simulink model "RobotModel6"  (R2025b)
settings: Solver=VariableStepAuto  StartTime=0.0  StopTime=100  RelTol=0.01  AbsTol=0.01  EnableMultiTasking=on
values from neighbouring files (symbols this model uses):
  waypoints = [R*cos(theta)+5, R*sin(theta)]    [init_waypoints.m]
undefined symbols (not defined in the file or in its folder): X, Y, Z
libraries: sm_lib x76, nesl_utility x37, slpidlib x2, robotalgslib x1, sharedtransform x1
(part 4 of 4)

== system RobotModel6/Subsystem5 ==
  In2 : Inport
  wR_cmd : Inport  Port=2
  PID Controller : slpidlib/PID Controller  Controller=PID  Form=Parallel  TimeDomain=Continuous-time  UseExternalTs=off  SampleTime=-1  IntegratorMethod=Forward Euler  FilterMethod=Forward Euler  ControllerParametersSource=internal  P=5  I=0  UseKiTs=off  D=0  UseExternalDerivativeSource=off  N=100  UseFilter=on  TunerSelectOption=Transfer Function Based (PID Tuner App)  InitialConditionSource=internal  InitialConditionForIntegrator=0  InitialConditionForFilter=0  DifferentiatorICPrevScaledInput=0  ExternalReset=none  TrackingMode=off  Kt=1  LimitOutput=off  SatLimitsSource=internal  UpperSaturationLimit=inf  LowerSaturationLimit=-inf  LinearizeAsGain=on  AntiWindupMode=none  Kb=1  LimitIntegrator=off  UpperIntegratorSaturationLimit=inf  LowerIntegratorSaturationLimit=-inf  POutMin=[]  POutMax=[]  IOutMin=[]  IOutMax=[]  DOutMin=[]  DOutMax=[]  NOutMin=[]  NOutMax=[]  SumOutMin=[]  SumOutMax=[]  SaturationOutMin=[]  SaturationOutMax=[]  PParamMin=[]  PParamMax=[]  IParamMin=[]  IParamMax=[]  DParamMin=[]  DParamMax=[]  NParamMin=[]  NParamMax=[]  KbParamMin=[]  KbParamMax=[]  KtParamMin=[]  KtParamMax=[]  KbOutMin=[]  KbOutMax=[]  KtOutMin=[]  KtOutMax=[]  IntegratorOutMin=[]  IntegratorOutMax=[]  FilterOutMin=[]  FilterOutMax=[]  SumI1OutMin=[]  SumI1OutMax=[]  SumI2OutMin=[]  SumI2OutMax=[]  SumI3OutMin=[]  SumI3OutMax=[]  SumI4OutMin=[]  SumI4OutMax=[]  SumDOutMin=[]  SumDOutMax=[]  DifferentiatorOutMin=[]  DifferentiatorOutMax=[]  FilterDiffOutCoefMin=[]  FilterDiffOutCoefMax=[]  ReciprocalOutMin=[]  ReciprocalOutMax=[]  SumDenOutMin=[]  SumDenOutMax=[]  SumNumOutMin=[]  SumNumOutMax=[]  DivideOutMin=[]  DivideOutMax=[]  UdiffTsProdOutMin=[]  UdiffTsProdOutMax=[]  NTsProdOutMin=[]  NTsProdOutMax=[]  UintegralTsProdOutMin=[]  UintegralTsProdOutMax=[]  UngainTsProdOutMin=[]  UngainTsProdOutMax=[]  ClampingZeroOutDataTypeStr=Inherit: Inherit via back propagation  ClampingZeroOutMin=[]  ClampingZeroOutMax=[]  FilterDenConstantOutDataTypeStr=Inherit: Inherit via back propagation  FilterDenConstantOutMin=[]  FilterDenConstantOutMax=[]  PCopyOutDataTypeStr=Inherit: Inherit via back propagation  PCopyOutMin=[]  PCopyOutMax=[]  NCopyOutDataTypeStr=Inherit: Inherit via back propagation  NCopyOutMin=[]  NCopyOutMax=[]  IntegratorContinuousStateAttributes=''  IntegratorStateMustResolveToSignalObject=off  IntegratorRTWStateStorageClass=Auto  FilterContinuousStateAttributes=''  FilterStateMustResolveToSignalObject=off  FilterRTWStateStorageClass=Auto  ParallelPVariant=InternalParameters  IdealPVariant=Disabled  IVariant=InternalParameters  DVariant=InternalParameters  IntegratorVariant=Continuous  SatVariant=Disabled  AWVariant=Passthrough  PCopyVariant=Disabled  TRVariant=Disabled  FdbkBlocksVariant=Forward  IdealPFdbkVariant=Disabled  SatFdbkVariant=Disabled  DerivativeFilterVariant=ContFilter  NVariant=InternalParameters  NCopyVariant=Disabled  FilterICVariant=InternalICsFilter  IntegratorICVariant=InternalICs  ExternalResetVariant=Disabled  TRSumVariant=Passthrough  SumFdbkVariant=Disabled  SumVariant=Sum_PID  TsampFilterVariant=InternalTs  TsampNgainVariant=Passthrough  TsampIntegralVariant=Disabled_SignalSpec  ExternalSaturationOutDataTypeStr=Inherit: Same as second input  DerivativeSourceVariant=ErrorSignal  PreIntVariant=InternalPreInt
  Saturation : Saturate  UpperLimit=5  LowerLimit=-5
  Subtract : Sum  Inputs=+-
  Out1 : Outport
  wires:
  In2/1 -> Subtract/2
  Subtract/1 -> PID Controller/1
  Saturation/1 -> Out1/1
  PID Controller/1 -> Saturation/1
  wR_cmd/1 -> Subtract/1

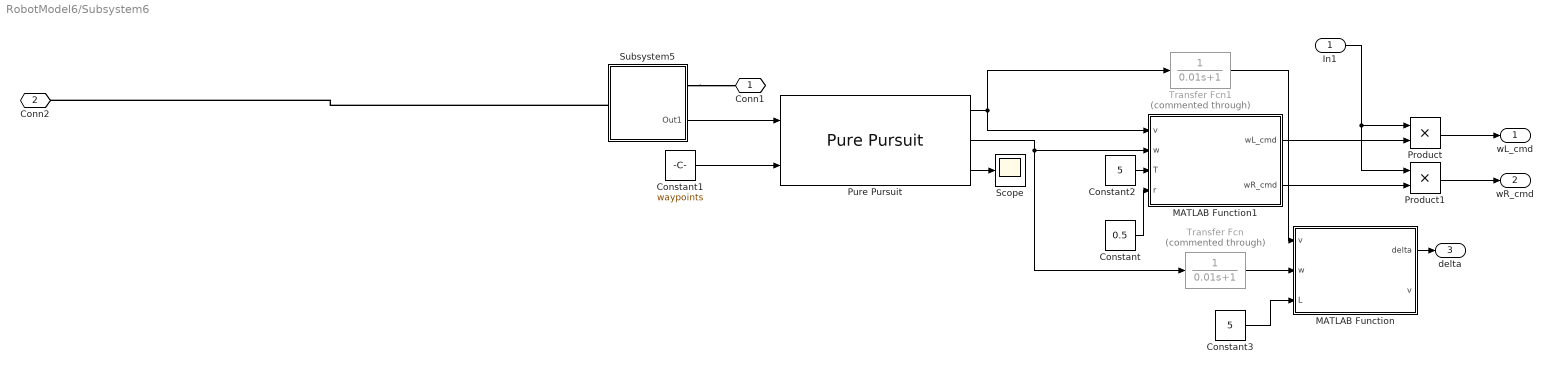
== system RobotModel6/Subsystem6 ==
  In1 : Inport
  Constant : Constant  Value=0.5
  Constant1 : Constant  Value=waypoints
  Constant2 : Constant  Value=5
  Constant3 : Constant  Value=5
  MATLAB Function : MATLAB Function  TreatAsAtomicUnit=on
  MATLAB Function1 : MATLAB Function  TreatAsAtomicUnit=on
  Product : Product
  Product1 : Product
  Pure Pursuit : robotalgslib/Pure Pursuit  DesiredLinearVelocityPort=off  DesiredLinearVelocity=6  MaxAngularVelocity=2  LookaheadDistancePort=off  LookaheadDistance=4  TargetDirPort=on  SimulateUsing=Code generation
      settings: LibrarySourceBlock=navlib/Control Algorithms/Pure Pursuit
  Scope : Scope
      settings: ActiveDisplayYMinimum=-4.8040636325719674  ActiveDisplayYMaximum=3.5962705540777251
  Subsystem5 : Subsystem
      settings: PortSchema="{\"entries\":[{\"content\":{\"sides\":[{\"content\":{\"connectorIds\":[\"LConn1\"]},\"type\":\"ConnectorPlacement.EquallySpacedRectSide\",\"uuid\":\"ddf93349-53d1-49a0-944e-d0734f46f29a\"},{\"content\":{\"connectorIds\":[\"RConn1\",\"Out1\"],\"side\":\"RIGHT\"},\"type\":\"ConnectorPlacement.EquallySpacedRectSide\",\"uuid\":\"41423d35-5168-4258-b195-077866701bba\"},{\"content\":{\"side\":\"TOP\"},\"type\":\"ConnectorPlacement.EquallySpacedRectSide\",\"uuid\":\"a64c51dc-c679-4f29-97b2-168705ea0e49\"}]},\"type\":\"ConnectorPlacement.EquallySpacedConnector\",\"uuid\":\"ed4aabc3-31ac-4b26-a964-31268bbe4985\"}],\"packageUris\":[\"http://schema.mathworks.com/mf0/Connector/R2020b\"],\"version\":\"1.0\"}"
  Transfer Fcn : TransferFcn  Commented=through  Denominator=[0.01 1]
  Transfer Fcn1 : TransferFcn  Commented=through  Denominator=[0.01 1]
  Conn1 : PMIOPort  Side=Right
  Conn2 : PMIOPort  Port=2  Side=Left
  wL_cmd : Outport
  wR_cmd : Outport  Port=2
  delta : Outport  Port=3
  wires:
  Pure Pursuit/2 -> MATLAB Function1/2(w), Transfer Fcn/1
  Transfer Fcn1/1 -> MATLAB Function/1("v ")
  Transfer Fcn/1 -> MATLAB Function/2(w)
  Constant1/1 -> Pure Pursuit/2
  MATLAB Function/1(delta) -> delta/1
  Constant/1 -> MATLAB Function1/4(r)
  Constant2/1 -> MATLAB Function1/3(T)
  Constant3/1 -> MATLAB Function/3(L)
  Pure Pursuit/1 -> MATLAB Function1/1(v), Transfer Fcn1/1
  Pure Pursuit/3 -> Scope/1
  Subsystem5/1(Out1) -> Pure Pursuit/1
  In1/1 -> Product/1, Product1/1
  MATLAB Function1/1(wL_cmd) -> Product/2
  Product/1 -> wL_cmd/1
  MATLAB Function1/2(wR_cmd) -> Product1/2
  Product1/1 -> wR_cmd/1
  connections:
  Subsystem5/RConn1 -- Conn1/RConn1
  Subsystem5/LConn1 -- Conn2/RConn1

== system RobotModel6/Subsystem7 ==
  wL_cmd : Inport
  In2 : Inport  Port=2
  PID Controller : slpidlib/PID Controller  Controller=PID  Form=Parallel  TimeDomain=Continuous-time  UseExternalTs=off  SampleTime=-1  IntegratorMethod=Forward Euler  FilterMethod=Forward Euler  ControllerParametersSource=internal  P=5  I=0  UseKiTs=off  D=0  UseExternalDerivativeSource=off  N=100  UseFilter=on  TunerSelectOption=Transfer Function Based (PID Tuner App)  InitialConditionSource=internal  InitialConditionForIntegrator=0  InitialConditionForFilter=0  DifferentiatorICPrevScaledInput=0  ExternalReset=none  TrackingMode=off  Kt=1  LimitOutput=off  SatLimitsSource=internal  UpperSaturationLimit=inf  LowerSaturationLimit=-inf  LinearizeAsGain=on  AntiWindupMode=none  Kb=1  LimitIntegrator=off  UpperIntegratorSaturationLimit=inf  LowerIntegratorSaturationLimit=-inf  POutMin=[]  POutMax=[]  IOutMin=[]  IOutMax=[]  DOutMin=[]  DOutMax=[]  NOutMin=[]  NOutMax=[]  SumOutMin=[]  SumOutMax=[]  SaturationOutMin=[]  SaturationOutMax=[]  PParamMin=[]  PParamMax=[]  IParamMin=[]  IParamMax=[]  DParamMin=[]  DParamMax=[]  NParamMin=[]  NParamMax=[]  KbParamMin=[]  KbParamMax=[]  KtParamMin=[]  KtParamMax=[]  KbOutMin=[]  KbOutMax=[]  KtOutMin=[]  KtOutMax=[]  IntegratorOutMin=[]  IntegratorOutMax=[]  FilterOutMin=[]  FilterOutMax=[]  SumI1OutMin=[]  SumI1OutMax=[]  SumI2OutMin=[]  SumI2OutMax=[]  SumI3OutMin=[]  SumI3OutMax=[]  SumI4OutMin=[]  SumI4OutMax=[]  SumDOutMin=[]  SumDOutMax=[]  DifferentiatorOutMin=[]  DifferentiatorOutMax=[]  FilterDiffOutCoefMin=[]  FilterDiffOutCoefMax=[]  ReciprocalOutMin=[]  ReciprocalOutMax=[]  SumDenOutMin=[]  SumDenOutMax=[]  SumNumOutMin=[]  SumNumOutMax=[]  DivideOutMin=[]  DivideOutMax=[]  UdiffTsProdOutMin=[]  UdiffTsProdOutMax=[]  NTsProdOutMin=[]  NTsProdOutMax=[]  UintegralTsProdOutMin=[]  UintegralTsProdOutMax=[]  UngainTsProdOutMin=[]  UngainTsProdOutMax=[]  ClampingZeroOutDataTypeStr=Inherit: Inherit via back propagation  ClampingZeroOutMin=[]  ClampingZeroOutMax=[]  FilterDenConstantOutDataTypeStr=Inherit: Inherit via back propagation  FilterDenConstantOutMin=[]  FilterDenConstantOutMax=[]  PCopyOutDataTypeStr=Inherit: Inherit via back propagation  PCopyOutMin=[]  PCopyOutMax=[]  NCopyOutDataTypeStr=Inherit: Inherit via back propagation  NCopyOutMin=[]  NCopyOutMax=[]  IntegratorContinuousStateAttributes=''  IntegratorStateMustResolveToSignalObject=off  IntegratorRTWStateStorageClass=Auto  FilterContinuousStateAttributes=''  FilterStateMustResolveToSignalObject=off  FilterRTWStateStorageClass=Auto  ParallelPVariant=InternalParameters  IdealPVariant=Disabled  IVariant=InternalParameters  DVariant=InternalParameters  IntegratorVariant=Continuous  SatVariant=Disabled  AWVariant=Passthrough  PCopyVariant=Disabled  TRVariant=Disabled  FdbkBlocksVariant=Forward  IdealPFdbkVariant=Disabled  SatFdbkVariant=Disabled  DerivativeFilterVariant=ContFilter  NVariant=InternalParameters  NCopyVariant=Disabled  FilterICVariant=InternalICsFilter  IntegratorICVariant=InternalICs  ExternalResetVariant=Disabled  TRSumVariant=Passthrough  SumFdbkVariant=Disabled  SumVariant=Sum_PID  TsampFilterVariant=InternalTs  TsampNgainVariant=Passthrough  TsampIntegralVariant=Disabled_SignalSpec  ExternalSaturationOutDataTypeStr=Inherit: Same as second input  DerivativeSourceVariant=ErrorSignal  PreIntVariant=InternalPreInt
  Saturation : Saturate  UpperLimit=5  LowerLimit=-5
  Subtract : Sum  Inputs=+-
  Out1 : Outport
  wires:
  In2/1 -> Subtract/2
  Subtract/1 -> PID Controller/1
  Saturation/1 -> Out1/1
  PID Controller/1 -> Saturation/1
  wL_cmd/1 -> Subtract/1

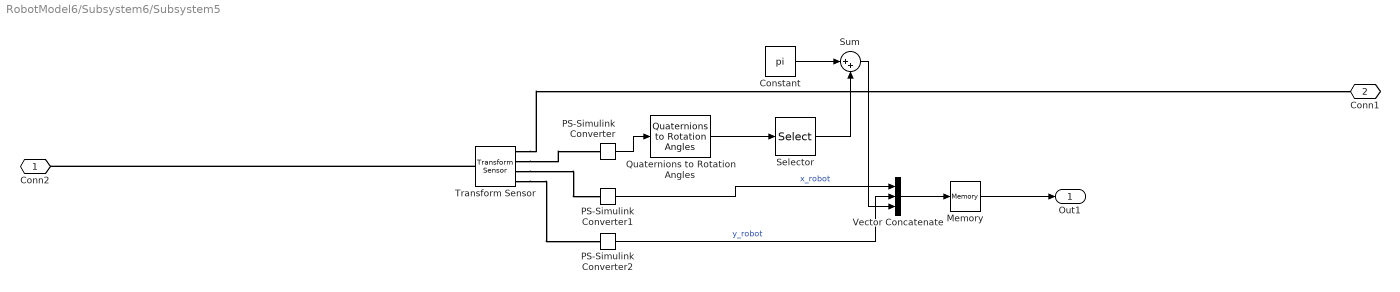
== system RobotModel6/Subsystem6/Subsystem5 ==
  Constant : Constant  Value=pi
  Memory : Memory
  PS-Simulink Converter : nesl_utility/PS-Simulink Converter  PhysicalDomain=network_engine_domain  SubClassName=ps_output  LeftPortType=input  RightPortType=output  PseudoPeriodic=off  Frequencies=[]  VectorFormat=inherit  Unit=inherit  AffineConversion=off
  PS-Simulink Converter1 : nesl_utility/PS-Simulink Converter  PhysicalDomain=network_engine_domain  SubClassName=ps_output  LeftPortType=input  RightPortType=output  PseudoPeriodic=off  Frequencies=[]  VectorFormat=inherit  Unit=inherit  AffineConversion=off
  PS-Simulink Converter2 : nesl_utility/PS-Simulink Converter  PhysicalDomain=network_engine_domain  SubClassName=ps_output  LeftPortType=input  RightPortType=output  PseudoPeriodic=off  Frequencies=[]  VectorFormat=inherit  Unit=inherit  AffineConversion=off
  Quaternions to Rotation Angles : sharedtransform/Quaternions to Rotation Angles  rotationOrder=ZYX  aMode=aMode
  Selector : Selector  InputPortWidth=3  IndexOptions=Index vector (dialog)  Indices=[1]  OutputSizes=1
  Sum : Sum  Inputs=|++
  Transform Sensor : sm_lib/Frames and Transforms/Transform Sensor  MeasurementFrame=World  RotationSequence=XYX  SenseAngle=off  SenseAxis=off  SenseQ=on  SenseR=off  SenseRotationSequence=off  SenseOmegaX=off  SenseOmegaY=off  SenseOmegaZ=off  SenseOmega=off  SenseQDot=off  SenseRDot=off  SenseRotationSequenceDot=off  SenseAlphaX=off  SenseAlphaY=off  SenseAlphaZ=off  SenseAlpha=off  SenseQDDot=off  SenseRDDot=off  SenseX=on  SenseY=on  SenseZ=off  SenseXYZ=off  SenseRad=off  SenseAzim=off  SenseDist=off  SenseInc=off  SenseXDot=off  SenseYDot=off  SenseZDot=off  SenseXYZDot=off  SenseRadDot=off  SenseAzimDot=off  SenseDistDot=off  SenseIncDot=off  SenseXDDot=off  SenseYDDot=off  SenseZDDot=off  SenseXYZDDot=off  SenseRadDDot=off  SenseAzimDDot=off  SenseDistDDot=off  SenseIncDDot=off
  Vector Concatenate : Concatenate  NumInputs=3
  Conn2 : PMIOPort  Side=Left
  Conn1 : PMIOPort  Port=2  Side=Right
  Out1 : Outport
  wires:
  Quaternions to Rotation Angles/1 -> Selector/1
  PS-Simulink Converter/1 -> Quaternions to Rotation Angles/1
  Vector Concatenate/1 -> Memory/1
  Memory/1 -> Out1/1
  PS-Simulink Converter1/1 -> Vector Concatenate/1  "x_robot"
  PS-Simulink Converter2/1 -> Vector Concatenate/2  "y_robot"
  Selector/1 -> Sum/2
  Constant/1 -> Sum/1
  Sum/1 -> Vector Concatenate/3
  connections:
  Transform Sensor/LConn1 -- Conn2/RConn1
  Transform Sensor/RConn4 -- PS-Simulink Converter2/LConn1
  Transform Sensor/RConn2 -- PS-Simulink Converter/LConn1
  Transform Sensor/RConn3 -- PS-Simulink Converter1/LConn1
  Transform Sensor/RConn1 -- Conn1/RConn1

== matlab function RobotModel6/RL/MATLAB Function1 ==
  data: mode_cmd input; alpha input; tau output; q input; dq input; q_cmd input; is_locked output; q_ref output
function [tau, is_locked, q_ref] = LockJointPD(mode_cmd, alpha, q, dq, q_cmd)
%#codegen
% mode_cmd: 0=Walk (track q_cmd), 1=Wheeled (lock current angle)
% alpha   : [0,1] smoothing factor (TransferFcn output), 0=fully walking, 1=fully locked
% q,dq    : joint angle/angular velocity
% q_cmd   : walk/stand target angle (radians)
Kp = 1200.0;   % Starting value, tune per joint
Kd =   20.0;
tau_lim = 300.0;
m = uint8(mode_cmd ~= 0);     % Standardize to uint8(0/1)
a = double(alpha);
persistent q_hold last_mode
if isempty(q_hold),    q_hold    = q;        end   % double
if isempty(last_mode), last_mode = uint8(0); end   % uint8
% Rising edge: 0->1, latch current angle
if (last_mode == uint8(0)) && (m ~= uint8(0))
    q_hold = q;
end
last_mode = m;
% Reference angle: interpolate between "hold angle" and "target angle"
q_ref  = a*q_hold + (1-a)*q_cmd;
dq_ref = 0.0;
% PD
tau = Kp*(q_ref - q) + Kd*(dq_ref - dq);
% Saturation
tau = max(min(tau, tau_lim), -tau_lim);
% Debug flag: is leg lock dominant
is_locked = (a > 0.5);     % Can also output m==1
end

== matlab function RobotModel6/Subsystem6/MATLAB Function1 ==
  data: v input; wL_cmd output; w input; T input; r input; wR_cmd output
function [wL_cmd, wR_cmd] = wheelSpeedCmd(v, w, T, r)
% v: linear velocity [m/s]
% w: 航向角速度 [rad/s]
% T: 后轮距 [m]
% r: 车轮半径 [m]

vL = v - 0.5*T*w;
vR = v + 0.5*T*w;

wL_cmd = vL / r;
wR_cmd = vR / r;
end

== matlab function RobotModel6/Subsystem6/MATLAB Function ==
  data: v input; delta output; w input; L input; v output
function [delta, v] = Diff2Ackermann(v, w, L)
% input: 
%   v - Linear velocity (m/s)
%   w - Angular velocity (rad/s)
%   L -  (m)
%
% output:
%   delta - front wheel rotation angel (rad)
%   v     -  velocity(m/s)
if abs(v) < 1e-3
    delta = 0;
else
    delta = atan(L * w / v);   % pure pursuit function
end

== matlab function RobotModel6/RR_climb/MATLAB Function ==
  data: t input; q output; mode_cmd input
function q = knee_FL_motion(t, mode_cmd)
%#codegen

Tsw = 70;   % 切换时间

% ------- 轮式模式：锁住，腿不动 -------
if (mode_cmd == 1) || (t < Tsw)
    q = 0;          % 回到原位（站立角）
    return;
end

% ------- 腿式模式：先蹲再站 -------
tau = t - Tsw;      % 本地时间

% 对应髋关节的三个阶段：T1 蹲下，T2 保持，T3 站起
T1 = 3;    % 蹲下用时
T2 = 15;    % 低姿态保持时间
T3 = 3;    % 站起用时

% 膝关节的站立角和蹲下角
q_stand = 0;                % 站立时膝盖角（回原位就是这个）
q_squat = deg2rad(70);      % 蹲下时膝盖最大弯曲

% --- 段1：从站立 -> 蹲下 ---
if tau < T1
    u = tau / T1;                           % 0→1
    q = (1-u)*q_stand + u*q_squat;

% --- 段2：保持蹲下姿态 ---
elseif tau < T1 + T2
    q = q_squat;

% --- 段3：从蹲下 -> 回到原位 ---
elseif tau < T1 + T2 + T3
    u = (tau - (T1 + T2)) / T3;
    q = (1-u)*q_squat + u*q_stand;

% --- 结束后一直保持原位 ---
else
    q = q_stand;
end
end

== matlab function RobotModel6/FR_climb/MATLAB Function2 ==
  data: t input; q output; mode_cmd input
function q = knee_FL_motion(t, mode_cmd)
%#codegen

Tsw = 70;   % 切换时间

% ------- 轮式模式：锁住，腿不动 -------
if (mode_cmd == 1) || (t < Tsw)
    q = 0;          % 回到原位（站立角）
    return;
end

% ------- 腿式模式：先蹲再站 -------
tau = t - Tsw;      % 本地时间

% 对应髋关节的三个阶段：T1 蹲下，T2 保持，T3 站起
T1 = 3;    % 蹲下用时
T2 = 15;    % 低姿态保持时间
T3 = 3;    % 站起用时

% 膝关节的站立角和蹲下角
q_stand = 0;                % 站立时膝盖角（回原位就是这个）
q_squat = deg2rad(70);      % 蹲下时膝盖最大弯曲

% --- 段1：从站立 -> 蹲下 ---
if tau < T1
    u = tau / T1;                           % 0→1
    q = (1-u)*q_stand + u*q_squat;

% --- 段2：保持蹲下姿态 ---
elseif tau < T1 + T2
    q = q_squat;

% --- 段3：从蹲下 -> 回到原位 ---
elseif tau < T1 + T2 + T3
    u = (tau - (T1 + T2)) / T3;
    q = (1-u)*q_squat + u*q_stand;

% --- 结束后一直保持原位 ---
else
    q = q_stand;
end
end

== matlab function RobotModel6/RL_climb/MATLAB Function ==
  data: t input; q output; mode_cmd input
function q = knee_FL_motion(t, mode_cmd)
%#codegen

Tsw = 70;   % 切换时间

% ------- 轮式模式：锁住，腿不动 -------
if (mode_cmd == 1) || (t < Tsw)
    q = 0;          % 回到原位（站立角）
    return;
end

% ------- 腿式模式：先蹲再站 -------
tau = t - Tsw;      % 本地时间

% 对应髋关节的三个阶段：T1 蹲下，T2 保持，T3 站起
T1 = 3;    % 蹲下用时
T2 = 15;    % 低姿态保持时间
T3 = 3;    % 站起用时

% 膝关节的站立角和蹲下角
q_stand = 0;                % 站立时膝盖角（回原位就是这个）
q_squat = deg2rad(70);      % 蹲下时膝盖最大弯曲

% --- 段1：从站立 -> 蹲下 ---
if tau < T1
    u = tau / T1;                           % 0→1
    q = (1-u)*q_stand + u*q_squat;

% --- 段2：保持蹲下姿态 ---
elseif tau < T1 + T2
    q = q_squat;

% --- 段3：从蹲下 -> 回到原位 ---
elseif tau < T1 + T2 + T3
    u = (tau - (T1 + T2)) / T3;
    q = (1-u)*q_squat + u*q_stand;

% --- 结束后一直保持原位 ---
else
    q = q_stand;
end
end

== matlab function RobotModel6/RL/MATLAB Function3 ==
  data: brake_en input; tau output; w input
function tau = BrakeTorque(brake_en, w)
%#codegen
% brake_en: 0=不刹车, 1=开始刹车
% w: 轮子角速度 (rad/s)，来自 Revolute Joint 的 Velocity 输出

Kb = 30.0;       % 阻尼系数，越大刹车越狠，可调
tau_max = 150.0; % 最大刹车扭矩限幅
w_eps = 0.05;    % 认为“已经停下”的速度阈值

if brake_en == 0
    tau = 0.0;     % 不刹车
    return;
end

% 速度很小就不再给力，避免抖动
if abs(w) < w_eps
    tau = 0.0;
else
    % 阻尼刹车：扭矩方向与角速度相反
    tau = -Kb * w;
end

% 扭矩限幅
if tau >  tau_max, tau =  tau_max; end
if tau < -tau_max, tau = -tau_max; end
end

== matlab function RobotModel6/RR/MATLAB Function1 ==
  data: mode_cmd input; alpha input; tau output; q input; dq input; q_cmd input; is_locked output; q_ref output
function [tau, is_locked, q_ref] = LockJointPD(mode_cmd, alpha, q, dq, q_cmd)
%#codegen
% mode_cmd: 0=Walk (track q_cmd), 1=Wheeled (lock current angle)
% alpha   : [0,1] smoothing factor (TransferFcn output), 0=fully walking, 1=fully locked
% q,dq    : joint angle/angular velocity
% q_cmd   : walk/stand target angle (radians)
Kp = 1200.0;   % Starting value, tune per joint
Kd =   20.0;
tau_lim = 300.0;
m = uint8(mode_cmd ~= 0);     % Standardize to uint8(0/1)
a = double(alpha);
persistent q_hold last_mode
if isempty(q_hold),    q_hold    = q;        end   % double
if isempty(last_mode), last_mode = uint8(0); end   % uint8
% Rising edge: 0->1, latch current angle
if (last_mode == uint8(0)) && (m ~= uint8(0))
    q_hold = q;
end
last_mode = m;
% Reference angle: interpolate between "hold angle" and "target angle"
q_ref  = a*q_hold + (1-a)*q_cmd;
dq_ref = 0.0;
% PD
tau = Kp*(q_ref - q) + Kd*(dq_ref - dq);
% Saturation
tau = max(min(tau, tau_lim), -tau_lim);
% Debug flag: is leg lock dominant
is_locked = (a > 0.5);     % Can also output m==1
end

== matlab function RobotModel6/RR/MATLAB Function2 ==
  data: t input; w output
function w = wheel_speed(t)
%#codegen

Tsw = 68;          % 开始动
Tacc = 2;          % 加速时间
V = 100;           % 最终匀速

if t < Tsw
    w = 0;

elseif t < Tsw + Tacc
    u = (t - Tsw) / Tacc;   % 0→1
    w = u * V;              % 线性从0加到V

else
    w = V;                  % 匀速巡航
end
end

== matlab function RobotModel6/RL/MATLAB Function2 ==
  data: t input; w output
function w = wheel_speed(t)
%#codegen

Tsw = 68;          % 开始动
Tacc = 2;          % 加速时间
V = 100;           % 最终匀速

if t < Tsw
    w = 0;

elseif t < Tsw + Tacc
    u = (t - Tsw) / Tacc;   % 0→1
    w = u * V;              % 线性从0加到V

else
    w = V;                  % 匀速巡航
end
end

== matlab function RobotModel6/FL_climb/MATLAB Function1 ==
  data: t input; q output; mode_cmd input
function q = knee_FL_motion(t, mode_cmd)
%#codegen

Tsw = 70;   % 切换时间

% ------- 轮式模式：锁住，腿不动 -------
if (mode_cmd == 1) || (t < Tsw)
    q = 0;          % 回到原位（站立角）
    return;
end

% ------- 腿式模式：先蹲再站 -------
tau = t - Tsw;      % 本地时间

% 对应髋关节的三个阶段：T1 蹲下，T2 保持，T3 站起
T1 = 3;    % 蹲下用时
T2 = 15;    % 低姿态保持时间
T3 = 3;    % 站起用时

% 膝关节的站立角和蹲下角
q_stand = 0;                % 站立时膝盖角（回原位就是这个）
q_squat = deg2rad(70);      % 蹲下时膝盖最大弯曲

% --- 段1：从站立 -> 蹲下 ---
if tau < T1
    u = tau / T1;                           % 0→1
    q = (1-u)*q_stand + u*q_squat;

% --- 段2：保持蹲下姿态 ---
elseif tau < T1 + T2
    q = q_squat;

% --- 段3：从蹲下 -> 回到原位 ---
elseif tau < T1 + T2 + T3
    u = (tau - (T1 + T2)) / T3;
    q = (1-u)*q_squat + u*q_stand;

% --- 结束后一直保持原位 ---
else
    q = q_stand;
end
end

== matlab function RobotModel6/FR_climb/MATLAB Function3 ==
  data: t input; q output; mode_cmd input
function q = hip_FL_motion(t, mode_cmd)
%#codegen

Tsw = 70;

% 轮式阶段：髋关节锁在 0
if (mode_cmd == 1) || (t < Tsw)
    q = 0;          % 轮式时锁住髋关节
    return;
end

% 腿式阶段：开始做“先蹲后站”的动作
tau = t - Tsw;      % 本地时间，从切换时刻重新计

% 姿态角（单位：rad）
q_stand = 0;                  % 站立时髋角
q_squat = -deg2rad(35);       % 蹲下时髋角（负是往上收腿）
% 你觉得不够矮可以再调大一点绝对值，比如 -45°

% 时间设置（和膝盖可以对应着来）
T1 = 3;    % 蹲下用时
T2 = 15;    % 低姿态保持时间
T3 = 3;    % 站起来用时
% 总时长 T1+T2+T3 之后保持站立

% --- 段1：从站立 -> 蹲下 ---
if tau < T1
    u = tau / T1;                      % 0→1
    q = (1-u)*q_stand + u*q_squat;

% --- 段2：保持蹲下姿态 ---
elseif tau < T1 + T2
    q = q_squat;

% --- 段3：从蹲下 -> 站回原位 ---
elseif tau < T1 + T2 + T3
    u = (tau - (T1 + T2)) / T3;
    q = (1-u)*q_squat + u*q_stand;

% --- 结束后：保持站立 ---
else
    q = q_stand;
end
end

== matlab function RobotModel6/RL_climb/MATLAB Function1 ==
  data: t input; q output; mode_cmd input
function q = hip_FL_motion(t, mode_cmd)
%#codegen

Tsw = 70;

% 轮式阶段：髋关节锁在 0
if (mode_cmd == 1) || (t < Tsw)
    q = 0;          % 轮式时锁住髋关节
    return;
end

% 腿式阶段：开始做“先蹲后站”的动作
tau = t - Tsw;      % 本地时间，从切换时刻重新计

% 姿态角（单位：rad）
q_stand = 0;                  % 站立时髋角
q_squat = -deg2rad(35);       % 蹲下时髋角（负是往上收腿）
% 你觉得不够矮可以再调大一点绝对值，比如 -45°

% 时间设置（和膝盖可以对应着来）
T1 = 3;    % 蹲下用时
T2 = 15;    % 低姿态保持时间
T3 = 3;    % 站起来用时
% 总时长 T1+T2+T3 之后保持站立

% --- 段1：从站立 -> 蹲下 ---
if tau < T1
    u = tau / T1;                      % 0→1
    q = (1-u)*q_stand + u*q_squat;

% --- 段2：保持蹲下姿态 ---
elseif tau < T1 + T2
    q = q_squat;

% --- 段3：从蹲下 -> 站回原位 ---
elseif tau < T1 + T2 + T3
    u = (tau - (T1 + T2)) / T3;
    q = (1-u)*q_squat + u*q_stand;

% --- 结束后：保持站立 ---
else
    q = q_stand;
end
end

== matlab function RobotModel6/RR_climb/MATLAB Function1 ==
  data: t input; q output; mode_cmd input
function q = hip_FL_motion(t, mode_cmd)
%#codegen

Tsw = 68;

% 轮式阶段：髋关节锁在 0
if (mode_cmd == 1) || (t < Tsw)
    q = 0;          % 轮式时锁住髋关节
    return;
end

% 腿式阶段：开始做“先蹲后站”的动作
tau = t - Tsw;      % 本地时间，从切换时刻重新计

% 姿态角（单位：rad）
q_stand = 0;                  % 站立时髋角
q_squat = -deg2rad(35);       % 蹲下时髋角（负是往上收腿）

% 时间设置（和膝盖可以对应着来）
T1 = 3;    % 蹲下用时
T2 = 15;    % 低姿态保持时间
T3 = 3;    % 站起来用时
% 总时长 T1+T2+T3 之后保持站立

% --- 段1：从站立 -> 蹲下 ---
if tau < T1
    u = tau / T1;                      % 0→1
    q = (1-u)*q_stand + u*q_squat;

% --- 段2：保持蹲下姿态 ---
elseif tau < T1 + T2
    q = q_squat;

% --- 段3：从蹲下 -> 站回原位 ---
elseif tau < T1 + T2 + T3
    u = (tau - (T1 + T2)) / T3;
    q = (1-u)*q_squat + u*q_stand;

% --- 结束后：保持站立 ---
else
    q = q_stand;
end
end

== matlab function RobotModel6/RR/MATLAB Function3 ==
  data: brake_en input; tau output; w input
function tau = BrakeTorque(brake_en, w)
%#codegen
% brake_en: 0=不刹车, 1=开始刹车
% w: 轮子角速度 (rad/s)，来自 Revolute Joint 的 Velocity 输出

Kb = 30.0;       % 阻尼系数，越大刹车越狠，可调
tau_max = 150.0; % 最大刹车扭矩限幅
w_eps = 0.05;    % 认为“已经停下”的速度阈值

if brake_en == 0
    tau = 0.0;     % 不刹车
    return;
end

% 速度很小就不再给力，避免抖动
if abs(w) < w_eps
    tau = 0.0;
else
    % 阻尼刹车：扭矩方向与角速度相反
    tau = -Kb * w;
end

% 扭矩限幅
if tau >  tau_max, tau =  tau_max; end
if tau < -tau_max, tau = -tau_max; end
end

== matlab function RobotModel6/FL_climb/MATLAB Function4 ==
  data: t input; q output; mode_cmd input
function q = hip_FL_motion(t, mode_cmd)
%#codegen

Tsw = 68;

% 轮式阶段：髋关节锁在 0
if (mode_cmd == 1) || (t < Tsw)
    q = 0;          % 轮式时锁住髋关节
    return;
end

% 腿式阶段：开始做“先蹲后站”的动作
tau = t - Tsw;      % 本地时间，从切换时刻重新计

% 姿态角（单位：rad）
q_stand = 0;                  % 站立时髋角
q_squat = -deg2rad(35);       % 蹲下时髋角（负是往上收腿）

% 时间设置（和膝盖可以对应着来）
T1 = 3;    % 蹲下用时
T2 = 15;    % 低姿态保持时间
T3 = 3;    % 站起来用时
% 总时长 T1+T2+T3 之后保持站立

% --- 段1：从站立 -> 蹲下 ---
if tau < T1
    u = tau / T1;                      % 0→1
    q = (1-u)*q_stand + u*q_squat;

% --- 段2：保持蹲下姿态 ---
elseif tau < T1 + T2
    q = q_squat;

% --- 段3：从蹲下 -> 站回原位 ---
elseif tau < T1 + T2 + T3
    u = (tau - (T1 + T2)) / T3;
    q = (1-u)*q_squat + u*q_stand;

% --- 结束后：保持站立 ---
else
    q = q_stand;
end
end

== matlab function RobotModel6/RR/MATLAB Function ==
  data: mode_cmd input; alpha input; tau output; q input; dq input; q_cmd input; is_locked output; q_ref output
function [tau, is_locked, q_ref] = LockJointPD(mode_cmd, alpha, q, dq, q_cmd)
%#codegen
% mode_cmd: 0=Walk(folloew q_cmd), 1=Wheel(lock the present angle )
% alpha   : [0,1] flatten faktor(TransferFcnoutput)，0=walk, 1=leg locked
% q,dq    : joint angle/angular velocity
% q_cmd   : walking/standing angle(rad)

Kp = 1200.0;   % start value
Kd =   20.0;
tau_lim = 300.0;

m = uint8(mode_cmd ~= 0);     % uint8(0/1)
a = double(alpha);

persistent q_hold last_mode
if isempty(q_hold),    q_hold    = q;        end   % double
if isempty(last_mode), last_mode = uint8(0); end   % uint8

% step: 0->1 
if (last_mode == uint8(0)) && (m ~= uint8(0))
    q_hold = q;
end
last_mode = m;

% reference angle
q_ref  = a*q_hold + (1-a)*q_cmd;
dq_ref = 0.0;

% PD
tau = Kp*(q_ref - q) + Kd*(dq_ref - dq);

% 
tau = max(min(tau, tau_lim), -tau_lim);

% 
is_locked = (a > 0.5);     % 
end

== matlab function RobotModel6/FR/MATLAB Function ==
  data: mode_cmd input; alpha input; tau output; q input; dq input; q_cmd input; is_locked output; q_ref output
function [tau, is_locked, q_ref] = LockJointPD(mode_cmd, alpha, q, dq, q_cmd)
%#codegen
% mode_cmd: 0=Walk (track q_cmd), 1=Wheeled (lock current angle)
% alpha   : [0,1] smoothing factor (TransferFcn output), 0=fully walking, 1=fully locked
% q,dq    : joint angle/angular velocity
% q_cmd   : walk/stand target angle (radians)
Kp = 1200.0;   % Starting value, tune per joint
Kd =   20.0;
tau_lim = 300.0;
m = uint8(mode_cmd ~= 0);     % Standardize to uint8(0/1)
a = double(alpha);
persistent q_hold last_mode
if isempty(q_hold),    q_hold    = q;        end   % double
if isempty(last_mode), last_mode = uint8(0); end   % uint8
% Rising edge: 0->1, latch current angle
if (last_mode == uint8(0)) && (m ~= uint8(0))
    q_hold = q;
end
last_mode = m;
% Reference angle: interpolate between "hold angle" and "target angle"
q_ref  = a*q_hold + (1-a)*q_cmd;
dq_ref = 0.0;
% PD
tau = Kp*(q_ref - q) + Kd*(dq_ref - dq);
% Saturation
tau = max(min(tau, tau_lim), -tau_lim);
% Debug flag: is leg lock dominant
is_locked = (a > 0.5);     % Can also output m==1
end

== matlab function RobotModel6/FR/MATLAB Function1 ==
  data: mode_cmd input; alpha input; tau output; q input; dq input; q_cmd input; is_locked output; q_ref output
function [tau, is_locked, q_ref] = LockJointPD(mode_cmd, alpha, q, dq, q_cmd)
%#codegen
% mode_cmd: 0=Walk (track q_cmd), 1=Wheeled (lock current angle)
% alpha   : [0,1] smoothing factor (TransferFcn output), 0=fully walking, 1=fully locked
% q,dq    : joint angle/angular velocity
% q_cmd   : walk/stand target angle (radians)
Kp = 1200.0;   % Starting value, tune per joint
Kd =   20.0;
tau_lim = 300.0;
m = uint8(mode_cmd ~= 0);     % Standardize to uint8(0/1)
a = double(alpha);
persistent q_hold last_mode
if isempty(q_hold),    q_hold    = q;        end   % double
if isempty(last_mode), last_mode = uint8(0); end   % uint8
% Rising edge: 0->1, latch current angle
if (last_mode == uint8(0)) && (m ~= uint8(0))
    q_hold = q;
end
last_mode = m;
% Reference angle: interpolate between "hold angle" and "target angle"
q_ref  = a*q_hold + (1-a)*q_cmd;
dq_ref = 0.0;
% PD
tau = Kp*(q_ref - q) + Kd*(dq_ref - dq);
% Saturation
tau = max(min(tau, tau_lim), -tau_lim);
% Debug flag: is leg lock dominant
is_locked = (a > 0.5);     % Can also output m==1
end

== matlab function RobotModel6/FL/MATLAB Function ==
  data: mode_cmd input; alpha input; tau output; q input; dq input; q_cmd input; is_locked output; q_ref output
function [tau, is_locked, q_ref] = LockJointPD(mode_cmd, alpha, q, dq, q_cmd)
%#codegen
% mode_cmd: 0=Walk (track q_cmd), 1=Wheeled (lock current angle)
% alpha   : [0,1] smoothing factor (TransferFcn output), 0=fully walking, 1=fully locked
% q,dq    : joint angle/angular velocity
% q_cmd   : walk/stand target angle (radians)
Kp = 1200.0;   % Starting value, tune per joint
Kd =   20.0;
tau_lim = 300.0;
m = uint8(mode_cmd ~= 0);     % Standardize to uint8(0/1)
a = double(alpha);
persistent q_hold last_mode
if isempty(q_hold),    q_hold    = q;        end   % double
if isempty(last_mode), last_mode = uint8(0); end   % uint8
% Rising edge: 0->1, latch current angle
if (last_mode == uint8(0)) && (m ~= uint8(0))
    q_hold = q;
end
last_mode = m;
% Reference angle: interpolate between "hold angle" and "target angle"
q_ref  = a*q_hold + (1-a)*q_cmd;
dq_ref = 0.0;
% PD
tau = Kp*(q_ref - q) + Kd*(dq_ref - dq);
% Saturation
tau = max(min(tau, tau_lim), -tau_lim);
% Debug flag: is leg lock dominant
is_locked = (a > 0.5);     % Can also output m==1
end

== matlab function RobotModel6/FL/MATLAB Function1 ==
  data: mode_cmd input; alpha input; tau output; q input; dq input; q_cmd input; is_locked output; q_ref output
function [tau, is_locked, q_ref] = LockJointPD(mode_cmd, alpha, q, dq, q_cmd)
%#codegen
% mode_cmd: 0=Walk (track q_cmd), 1=Wheeled (lock current angle)
% alpha   : [0,1] smoothing factor (TransferFcn output), 0=fully walking, 1=fully locked
% q,dq    : joint angle/angular velocity
% q_cmd   : walk/stand target angle (radians)
Kp = 1200.0;   % Starting value, tune per joint
Kd =   20.0;
tau_lim = 300.0;
m = uint8(mode_cmd ~= 0);     % Standardize to uint8(0/1)
a = double(alpha);
persistent q_hold last_mode
if isempty(q_hold),    q_hold    = q;        end   % double
if isempty(last_mode), last_mode = uint8(0); end   % uint8
% Rising edge: 0->1, latch current angle
if (last_mode == uint8(0)) && (m ~= uint8(0))
    q_hold = q;
end
last_mode = m;
% Reference angle: interpolate between "hold angle" and "target angle"
q_ref  = a*q_hold + (1-a)*q_cmd;
dq_ref = 0.0;
% PD
tau = Kp*(q_ref - q) + Kd*(dq_ref - dq);
% Saturation
tau = max(min(tau, tau_lim), -tau_lim);
% Debug flag: is leg lock dominant
is_locked = (a > 0.5);     % Can also output m==1
end

== matlab function RobotModel6/RL/MATLAB Function ==
  data: mode_cmd input; alpha input; tau output; q input; dq input; q_cmd input; is_locked output; q_ref output
function [tau, is_locked, q_ref] = LockJointPD(mode_cmd, alpha, q, dq, q_cmd)
%#codegen
% mode_cmd: 0=Walk (track q_cmd), 1=Wheeled (lock current angle)
% alpha   : [0,1] smoothing factor (TransferFcn output), 0=fully walking, 1=fully locked
% q,dq    : joint angle/angular velocity
% q_cmd   : walk/stand target angle (radians)
Kp = 1200.0;   % Starting value, tune per joint
Kd =   20.0;
tau_lim = 300.0;
m = uint8(mode_cmd ~= 0);     % Standardize to uint8(0/1)
a = double(alpha);
persistent q_hold last_mode
if isempty(q_hold),    q_hold    = q;        end   % double
if isempty(last_mode), last_mode = uint8(0); end   % uint8
% Rising edge: 0->1, latch current angle
if (last_mode == uint8(0)) && (m ~= uint8(0))
    q_hold = q;
end
last_mode = m;
% Reference angle: interpolate between "hold angle" and "target angle"
q_ref  = a*q_hold + (1-a)*q_cmd;
dq_ref = 0.0;
% PD
tau = Kp*(q_ref - q) + Kd*(dq_ref - dq);
% Saturation
tau = max(min(tau, tau_lim), -tau_lim);
% Debug flag: is leg lock dominant
is_locked = (a > 0.5);     % Can also output m==1
end
